simulink model "HVModAL_Fahrzeugmodell"  (R2015b)
settings: Solver=ode1  StartTime=0  StopTime=drp.driving_cycle.tstop  FixedStep=sim_params.Ts  RelTol=1e-5
PreLoadFcn:
  | % Add paths
  | addpath data
  | addpath(genpath('library'))
StartFcn:
  | Simulation.StartTime = tic;
StopFcn:
  | Simulation.DurationTime = toc(Simulation.StartTime);
undefined symbols (not defined in the file or in its folder): Batteries, BMS, BMS_Bat_, C_Nenn_DCDC1, C_Nenn_DCDC2, d2d, DC, DCDC_Converter_efficiency, DcDc_Converters, Dcl, drp, drv, elm, gen, gin, Hdc, hdc, HV, hvb, Hvb, ice, ldc, lib_dcl, lib_hdc, lib_hvb, lib_veh, Link, lossestable, mask_LUT_OCV, mask_LUT_OCV_SOC, mask_LUT_OCV_Temperature, mask_LUT_R, mask_LUT_Rs, mask_LUT_Rs_SOC, mask_LUT_Rs_Temperature, sim_params, speedvec, torquevec, tri, veh, Veh, Vehicle_Chassis
libraries: simulink x29, lib_tri_modules x7, lib_hdc_module x5, lib_gearbox x4, lib_hvb_battery_pack x3, cstblocks x3, PowerLimitBlock x2, MultiCellLibrary x2, lib_aux x1, lib_drv x1, lib_gen x1, lib_elm x1
(part 6 of 7)

== system HVModAL_Fahrzeugmodell/Energy Manager (Emg)/Battery Control/Driving_Mode/Strategy_Maximiziation_Available_Batterypower/Choice_Algorithm ==
  b_Bat_available_b_Bat1 : Inport
  b_Bat_available_b_Bat2 : Inport  Port=2
  b_Bat_available_b_Bat3 : Inport  Port=3
  n_Bat_type_ID_Bat1 : Inport  Port=4
  n_Bat_type_ID_Bat2 : Inport  Port=5
  n_Bat_type_ID_Bat3 : Inport  Port=6
  1_eq_2 : RelationalOperator  Operator===  OutDataTypeStr=boolean
  1_eq_3 : RelationalOperator  Operator===  OutDataTypeStr=boolean
  1av_AND_2av_AND_3av_AND_1_eq_2_eq3 : Logic  Inputs=6  AllPortsSameDT=off  OutDataTypeStr=boolean
  1av_AND_2av_AND_3not_av_AND_1_eq_2 : Logic  Inputs=4  AllPortsSameDT=off  OutDataTypeStr=boolean
  1av_AND_2not_av_AND_3av_AND_1_eq_3 : Logic  Inputs=4  AllPortsSameDT=off  OutDataTypeStr=boolean
  1not_av_AND_2av_AND_3av_AND_2_eq_3 : Logic  Inputs=4  AllPortsSameDT=off  OutDataTypeStr=boolean
  2_eq_3 : RelationalOperator  Operator===  OutDataTypeStr=boolean
  Logical Operator : Logic  Operator=NOT  AllPortsSameDT=off  OutDataTypeStr=boolean
  Logical Operator1 : Logic  Operator=NOT  AllPortsSameDT=off  OutDataTypeStr=boolean
  Logical Operator2 : Logic  Operator=NOT  AllPortsSameDT=off  OutDataTypeStr=boolean
  Logical Operator3 : Logic  Operator=OR  Inputs=4  AllPortsSameDT=off  OutDataTypeStr=boolean
  b_Strategy_SOC_Equalization : Outport
  wires:
  Logical Operator3/1 -> b_Strategy_SOC_Equalization/1
  1av_AND_2not_av_AND_3av_AND_1_eq_3/1 -> Logical Operator3/3
  1av_AND_2av_AND_3not_av_AND_1_eq_2/1 -> Logical Operator3/2
  1not_av_AND_2av_AND_3av_AND_2_eq_3/1 -> Logical Operator3/4
  1av_AND_2av_AND_3av_AND_1_eq_2_eq3/1 -> Logical Operator3/1
  Logical Operator2/1 -> 1not_av_AND_2av_AND_3av_AND_2_eq_3/1
  Logical Operator1/1 -> 1av_AND_2not_av_AND_3av_AND_1_eq_3/2
  Logical Operator/1 -> 1av_AND_2av_AND_3not_av_AND_1_eq_2/3
  1_eq_3/1 -> 1av_AND_2not_av_AND_3av_AND_1_eq_3/4, 1av_AND_2av_AND_3av_AND_1_eq_2_eq3/6
  2_eq_3/1 -> 1av_AND_2av_AND_3av_AND_1_eq_2_eq3/5, 1not_av_AND_2av_AND_3av_AND_2_eq_3/4
  1_eq_2/1 -> 1av_AND_2av_AND_3not_av_AND_1_eq_2/4, 1av_AND_2av_AND_3av_AND_1_eq_2_eq3/4
  n_Bat_type_ID_Bat3/1 -> 2_eq_3/2, 1_eq_3/2
  n_Bat_type_ID_Bat2/1 -> 1_eq_2/2, 2_eq_3/1
  n_Bat_type_ID_Bat1/1 -> 1_eq_2/1, 1_eq_3/1
  b_Bat_available_b_Bat3/1 -> Logical Operator/1, 1av_AND_2av_AND_3av_AND_1_eq_2_eq3/3, 1av_AND_2not_av_AND_3av_AND_1_eq_3/3, 1not_av_AND_2av_AND_3av_AND_2_eq_3/3
  b_Bat_available_b_Bat2/1 -> 1av_AND_2av_AND_3not_av_AND_1_eq_2/2, 1av_AND_2av_AND_3av_AND_1_eq_2_eq3/2, Logical Operator1/1, 1not_av_AND_2av_AND_3av_AND_2_eq_3/2
  b_Bat_available_b_Bat1/1 -> Logical Operator2/1, 1av_AND_2not_av_AND_3av_AND_1_eq_3/1, 1av_AND_2av_AND_3not_av_AND_1_eq_2/1, 1av_AND_2av_AND_3av_AND_1_eq_2_eq3/1

== system HVModAL_Fahrzeugmodell/Energy Manager (Emg)/Battery Control/Driving_Mode/Strategy_Maximiziation_Available_Batterypower/multiple_packs ==
  b_Bat_available_b_Bat1 : Inport
  b_Bat_available_b_Bat2 : Inport  Port=2
  b_Bat_available_b_Bat3 : Inport  Port=3
  Add : Sum  Inputs=+++
  Constant : Constant
  Display : Display
  Relational Operator : RelationalOperator  Operator=>  OutDataTypeStr=boolean
  b_MultiplePacks : Outport
  wires:
  b_Bat_available_b_Bat1/1 -> Add/1
  b_Bat_available_b_Bat2/1 -> Add/2
  b_Bat_available_b_Bat3/1 -> Add/3
  Add/1 -> Display/1, Relational Operator/1
  Constant/1 -> Relational Operator/2
  Relational Operator/1 -> b_MultiplePacks/1

== system HVModAL_Fahrzeugmodell/Energy Manager (Emg)/Battery Control/Driving_Mode/Strategy_Maximiziation_Available_Batterypower/only_one_Pack ==
  note: full power to available pack
  b_Bat_available_b_Bat1 : Inport
  b_Bat_available_b_Bat2 : Inport  Port=2
  b_Bat_available_b_Bat3 : Inport  Port=3
  Enable : EnablePort
  Gain : Gain  Gain=100
  Gain1 : Gain  Gain=100
  Gain2 : Gain  Gain=100
  Mux : Mux  Inputs=3
  vector_PowerDistribution : Outport
  wires:
  b_Bat_available_b_Bat1/1 -> Gain/1
  b_Bat_available_b_Bat2/1 -> Gain1/1
  b_Bat_available_b_Bat3/1 -> Gain2/1
  Mux/1 -> vector_PowerDistribution/1
  Gain/1 -> Mux/1
  Gain1/1 -> Mux/2
  Gain2/1 -> Mux/3

== system HVModAL_Fahrzeugmodell/Energy Manager (Emg)/Battery Control/Driving_Mode/Strategy_Maximiziation_Driving_Range1/Minloss Strategy ==
  SB_BMS_1 : Inport
  SB_BMS_2 : Inport  Port=2
  SB_BMS_3 : Inport  Port=3
  Pload : Inport  Port=4
  Bus Selector : BusSelector  OutputSignals=SOC_perc
  Compare To Constant : simulink/Logic and Bit Operations/Compare To Constant  relop=>=  const=20  OutDataTypeStr=boolean
  Insufficient Energy : Subsystem
  Logical Operator : Logic  Operator=NOT  AllPortsSameDT=off  OutDataTypeStr=boolean
  Merge : Merge
  Merge1 : Merge
  Sufficient Energy left : Subsystem
  vector_PowerDistribution : Outport
  P_exchange_Master_Slave : Outport  Port=2
  wires:
  Insufficient Energy/2(P_exchange_Master_Slave) -> Merge1/2
  Sufficient Energy left/2(P_exchange_Master_Slave) -> Merge1/1
  Merge1/1 -> P_exchange_Master_Slave/1
  Logical Operator/1 -> Insufficient Energy/Enable
  Merge/1 -> vector_PowerDistribution/1
  Insufficient Energy/1(vector_PowerDistribution) -> Merge/2
  Sufficient Energy left/1(vector_PowerDistribution) -> Merge/1
  Compare To Constant/1 -> Logical Operator/1, Sufficient Energy left/Enable
  Bus Selector/1 -> Compare To Constant/1  "<SOC_perc>"
  Pload/1 -> Sufficient Energy left/4(Pload), Insufficient Energy/4("Pload ")
  SB_BMS_3/1 -> Insufficient Energy/3("SB_BMS_3 "), Sufficient Energy left/3("SB_BMS_3 ")
  SB_BMS_2/1 -> Insufficient Energy/2(SB_BMS_2), Sufficient Energy left/2(SB_BMS_2)
  SB_BMS_1/1 -> Bus Selector/1, Insufficient Energy/1(SB_BMS_1), Sufficient Energy left/1(SB_BMS_1)

== system HVModAL_Fahrzeugmodell/Traction Inverters (Tri)/Tri1/Thermal Model/Conventional thermal model/Conventional thermal model ==
  P losses : Inport
  T_amb : Inport  Port=2
  Demux1 : Demux
  Mux3 : Mux
  Subsystem : Subsystem
  Temperature : Outport
  wires:
  Demux1/3 -> Subsystem/3(Ploss Ml)
  Demux1/2 -> Subsystem/2(Ploss Dh)
  Demux1/1 -> Subsystem/1(Ploss Mh)
  P losses/1 -> Demux1/1
  Demux1/4 -> Subsystem/4(Ploss Dl)
  T_amb/1 -> Subsystem/5(Water Temperature)
  Mux3/1 -> Temperature/1
  Subsystem/4(T Dl) -> Mux3/4
  Subsystem/3(T Ml) -> Mux3/3
  Subsystem/1(T Mh) -> Mux3/1
  Subsystem/2(T Dh) -> Mux3/2

== system HVModAL_Fahrzeugmodell/Traction Inverters (Tri)/Tri1/Thermal Model/Foster Model/Leg1 ==
  In1 : Inport
  Constant : Constant  Value=TRIname.ThermalModel.FosterModel.FosterModel.IGBT.firstValue
  Constant1 : Constant  Value=[TRIname.ThermalModel.FosterModel.FosterModel.Diode.firstValue]
  Constant2 : Constant  Value=[TRIname.ThermalModel.FosterModel.FosterModel.IGBT.firstValue]
  Constant3 : Constant  Value=[TRIname.ThermalModel.FosterModel.FosterModel.Diode.firstValue]
  Demux : Demux
  Mux : Mux
  Product{,1..3} (4 alike) : Product
  Sum{1..6,16,18} (8 alike) : Sum  Inputs=|++
  Transfer Fcn1 : TransferFcn  Numerator=[TRIname.ThermalModel.FosterModel.FosterModel.IGBT.secondValue]  Denominator=[TRIname.ThermalModel.FosterModel.FosterModel.IGBT.secondTau 1]
  Transfer Fcn2 : TransferFcn  Numerator=[TRIname.ThermalModel.FosterModel.FosterModel.IGBT.transientValue]  Denominator=[TRIname.ThermalModel.FosterModel.FosterModel.IGBT.transientTau 1]
  Transfer Fcn3 : TransferFcn  Numerator=[TRIname.ThermalModel.FosterModel.FosterModel.Diode.secondValue]  Denominator=[TRIname.ThermalModel.FosterModel.FosterModel.Diode.secondTau 1]
  Transfer Fcn4 : TransferFcn  Numerator=[TRIname.ThermalModel.FosterModel.FosterModel.Diode.transientValue]  Denominator=[TRIname.ThermalModel.FosterModel.FosterModel.Diode.transientTau 1]
  Transfer Fcn5 : TransferFcn  Numerator=[TRIname.ThermalModel.FosterModel.FosterModel.IGBT.secondValue]  Denominator=[TRIname.ThermalModel.FosterModel.FosterModel.IGBT.secondTau 1]
  Transfer Fcn6 : TransferFcn  Numerator=[TRIname.ThermalModel.FosterModel.FosterModel.IGBT.transientValue]  Denominator=[TRIname.ThermalModel.FosterModel.FosterModel.IGBT.transientTau 1]
  Transfer Fcn7 : TransferFcn  Numerator=[TRIname.ThermalModel.FosterModel.FosterModel.Diode.secondValue]  Denominator=[TRIname.ThermalModel.FosterModel.FosterModel.Diode.secondTau 1]
  Transfer Fcn8 : TransferFcn  Numerator=[TRIname.ThermalModel.FosterModel.FosterModel.Diode.transientValue]  Denominator=[TRIname.ThermalModel.FosterModel.FosterModel.Diode.transientTau 1]
  Leg1TempVec : Outport
  wires:
  Sum6/1 -> Mux/4
  Product2/1 -> Sum4/1
  Transfer Fcn5/1 -> Sum4/2
  Constant2/1 -> Product2/1
  Transfer Fcn8/1 -> Sum6/2
  Transfer Fcn7/1 -> Sum3/2
  Product3/1 -> Sum3/1
  Transfer Fcn6/1 -> Sum5/2
  Sum3/1 -> Sum6/1
  Sum4/1 -> Sum5/1
  Constant3/1 -> Product3/1
  Sum5/1 -> Mux/3
  Demux/3 -> Product2/2, Transfer Fcn5/1, Transfer Fcn6/1
  Demux/4 -> Transfer Fcn8/1, Transfer Fcn7/1, Product3/2
  Mux/1 -> Leg1TempVec/1
  In1/1 -> Demux/1
  Sum1/1 -> Sum2/1
  Demux/2 -> Product1/2, Transfer Fcn3/1, Transfer Fcn4/1
  Constant1/1 -> Product1/1
  Sum2/1 -> Mux/2
  Transfer Fcn4/1 -> Sum2/2
  Product1/1 -> Sum1/1
  Transfer Fcn3/1 -> Sum1/2
  Constant/1 -> Product/1
  Sum18/1 -> Mux/1
  Sum16/1 -> Sum18/1
  Demux/1 -> Transfer Fcn2/1, Transfer Fcn1/1, Product/2
  Transfer Fcn2/1 -> Sum18/2
  Product/1 -> Sum16/1
  Transfer Fcn1/1 -> Sum16/2

== system HVModAL_Fahrzeugmodell/Traction Inverters (Tri)/Tri1/Thermal Model old/Thermal Junction Model/Leg 1 ==
  In1 : Inport
  Leg 1_sfcn : S-Function  FunctionName=Leg_sf  SFunctionModules=""  SFunctionDeploymentMode=off  EnableBusSupport=off  mask{rtw_sf_name=Leg_sf, showVar=off}
      mask prompts: rtw_sf_name "Simulink:masks:GenSFuncName_MP"; showVar "Simulink:masks:GenSFuncShowModuleList_MP"
      mask help: Simulink:masks:GenSFuncDesc_MD
      mask init: same as HVModAL_Fahrzeugmodell/Energy Manager (Emg)/Battery Control1/Battery Control_sfcn
      settings: CopyFcn=|
      | if ~strcmp(get_param(gcb,'Linkstatus'),'none') && ...
      | ~strcmp(get_param(gcb,'Linkstatus'),'implicit')
      |   set_param(gcb,'LinkStatus','none');
      | end
      mask Help: eval('feval(''rtwprivate'',''rtwhelpview'',''rtw_sfcn_block'')');
      mask Display:
      | port_label('input',1,'In1');
      | port_label('output',1,'Out1');
  __InputSSForSFun__ : Subsystem
      settings: PermitHierarchicalResolution=ParametersOnly
  __OutputSSForSFun__ : Subsystem
      settings: PermitHierarchicalResolution=ParametersOnly
  Out1 : Outport  InitialOutput=0
  wires:
  __OutputSSForSFun__/1(Out1) -> Out1/1
  Leg 1_sfcn/1 -> __OutputSSForSFun__/1(__UniqueInportName__1__)
  __InputSSForSFun__/1(__UniqueOutportName__1__) -> Leg 1_sfcn/1
  In1/1 -> __InputSSForSFun__/1(In1)

== system HVModAL_Fahrzeugmodell/Traction Inverters (Tri)/Tri1/Thermal Model old/Thermal Junction Model/Leg 2 ==
  In1 : Inport
  Leg 1_sfcn : S-Function  FunctionName=Leg_sf  SFunctionModules=""  SFunctionDeploymentMode=off  EnableBusSupport=off  mask{rtw_sf_name=Leg_sf, showVar=off}
      mask prompts: rtw_sf_name "Simulink:masks:GenSFuncName_MP"; showVar "Simulink:masks:GenSFuncShowModuleList_MP"
      mask help: Simulink:masks:GenSFuncDesc_MD
      mask init: same as HVModAL_Fahrzeugmodell/Energy Manager (Emg)/Battery Control1/Battery Control_sfcn
      settings: CopyFcn=|
      | if ~strcmp(get_param(gcb,'Linkstatus'),'none') && ...
      | ~strcmp(get_param(gcb,'Linkstatus'),'implicit')
      |   set_param(gcb,'LinkStatus','none');
      | end
      mask Help: eval('feval(''rtwprivate'',''rtwhelpview'',''rtw_sfcn_block'')');
      mask Display:
      | port_label('input',1,'In1');
      | port_label('output',1,'Out1');
  __InputSSForSFun__ : Subsystem
      settings: PermitHierarchicalResolution=ParametersOnly
  __OutputSSForSFun__ : Subsystem
      settings: PermitHierarchicalResolution=ParametersOnly
  Out1 : Outport  InitialOutput=0
  wires:
  __OutputSSForSFun__/1(Out1) -> Out1/1
  Leg 1_sfcn/1 -> __OutputSSForSFun__/1(__UniqueInportName__1__)
  __InputSSForSFun__/1(__UniqueOutportName__1__) -> Leg 1_sfcn/1
  In1/1 -> __InputSSForSFun__/1(In1)

== system HVModAL_Fahrzeugmodell/Traction Inverters (Tri)/Tri1/Thermal Model old/Thermal Junction Model/Leg 3 ==
  In1 : Inport
  Leg 1_sfcn : S-Function  FunctionName=Leg_sf  SFunctionModules=""  SFunctionDeploymentMode=off  EnableBusSupport=off  mask{rtw_sf_name=Leg_sf, showVar=off}
      mask prompts: rtw_sf_name "Simulink:masks:GenSFuncName_MP"; showVar "Simulink:masks:GenSFuncShowModuleList_MP"
      mask help: Simulink:masks:GenSFuncDesc_MD
      mask init: same as HVModAL_Fahrzeugmodell/Energy Manager (Emg)/Battery Control1/Battery Control_sfcn
      settings: CopyFcn=|
      | if ~strcmp(get_param(gcb,'Linkstatus'),'none') && ...
      | ~strcmp(get_param(gcb,'Linkstatus'),'implicit')
      |   set_param(gcb,'LinkStatus','none');
      | end
      mask Help: eval('feval(''rtwprivate'',''rtwhelpview'',''rtw_sfcn_block'')');
      mask Display:
      | port_label('input',1,'In1');
      | port_label('output',1,'Out1');
  __InputSSForSFun__ : Subsystem
      settings: PermitHierarchicalResolution=ParametersOnly
  __OutputSSForSFun__ : Subsystem
      settings: PermitHierarchicalResolution=ParametersOnly
  Out1 : Outport  InitialOutput=0
  wires:
  In1/1 -> __InputSSForSFun__/1(In1)
  __InputSSForSFun__/1(__UniqueOutportName__1__) -> Leg 1_sfcn/1
  Leg 1_sfcn/1 -> __OutputSSForSFun__/1(__UniqueInportName__1__)
  __OutputSSForSFun__/1(Out1) -> Out1/1

== system HVModAL_Fahrzeugmodell/Energy Manager (Emg)/Battery Control/Driving_Mode/Range_extender 1/power_distribution_new/Subsystem ==
  note: #new#:
      | P_load-P_Bat2_max>0: --> P_load>P_Bat2_max --> P2=P_Bat2_max; P1=P_load-P2; discharge
      |
      | P_load-P_Bat2_max<0: --> 1): 0<P_load<P_Bat2_max -->P2=P_load*3; P1=P_load-P2; charged or (0<P_load<P_Bat2_max -->P2=P_load; P1=0;)
      |
      | 2): P_load<0 --> P2=|P_load|&P2<=P_Bat2_max; P1=P_load+P2; charged
  note: #previous#:
      | P_load-P_Bat2_max>0: --> P_load>P_Bat2_max --> P2=P_Bat2_max; P1=P_load-P2; discharge
      |
      | P_load-P_Bat2_max<0: --> 1): 0<P_load<P_Bat2_max -->P2=P_Bat2_max; P1=P_load-P2; charged
      |
      | 2): P_load<0 --> P2=P_Bat2_max; P1=P_load+P2; charged
  P_load : Inport
  P_Bat2_discharge_max : Inport  Port=2
  Constant1 : Constant  Value=0
  Gain : Gain  Gain=-1
  Gain1 : Gain  Gain=3
  P_Bat2_new : Scope  NumInputPorts=2
  P_Bat2_old : Scope  NumInputPorts=2
  P_UB_Bat1#2 : Scope
  Saturation1 : Saturate  UpperLimit=0  LowerLimit=-inf
  Subtract1 : Sum  Inputs=+-
  Subtract2 : Sum  Inputs=+-
  Subtract3 : Sum  Inputs=+-
  Switch{1,3..5} (4 alike) : Switch
  Switch2 : Switch  Threshold=5
  P_Bat2 : Outport
  wires:
  Switch1/1 -> P_Bat2/1, P_Bat2_new/2
  P_Bat2_discharge_max/1 -> Subtract2/2, Switch5/1, P_UB_Bat1#2/1, Switch1/1, Subtract3/2, Switch2/1
  Constant1/1 -> Switch2/3
  Switch2/1 -> Subtract1/2, Switch3/1
  Subtract1/1 -> Switch3/2
  Switch3/1 -> Switch4/1, Switch4/2
  Saturation1/1 -> Gain/1
  Gain/1 -> Switch5/3, Subtract2/1
  Subtract2/1 -> Switch5/2
  Switch5/1 -> Switch4/3
  Subtract3/1 -> Switch1/2
  Gain1/1 -> Switch1/3, Subtract3/1
  Switch4/1 -> P_Bat2_old/2, Gain1/1
  P_load/1 -> Switch2/2, Saturation1/1, Switch3/3, Subtract1/1, P_Bat2_new/1, P_Bat2_old/1

== system HVModAL_Fahrzeugmodell/Energy Manager (Emg)/Battery Control/Driving_Mode/Range_extender 2/dynamic/power estimination  ==
  note: pos. and negative
      | but != 0
  note: >0 --> Inverter take energy out of DC link (Acceleration)
      | <0 --> Inverter feed energy into DC link (Recuperation)
  note: calculate the voltage
  note: calculate the power
  P_max_Disch_W_Bat2 : Inport
  P_currentPower_W_Bat1 : Inport  Port=2
  P_currentPower_W_Bat2 : Inport  Port=3
  P_currentPower_W_Bat3 : Inport  Port=4
  P_max_ch_W_Bat1 : Inport  Port=5
  P_max_Disch_W_Bat1 : Inport  Port=6
  "I_rex " : Inport  Port=7
  P_currentPower_Inv_W : Inport  Port=8
  P_currentPower_Aux_W : Inport  Port=9
  Add1 : Sum
  Add2 : Sum  Inputs=+++
  Add3 : Sum
  Constant2 : Constant  Value=hvb.Bat2.cell.I_max_disch
  Constant3 : Constant  Value=0.1
  Divide1 : Product  Inputs=*/
  Gain : Gain  Gain=-1
  Gain1 : Gain
  Product1 : Product
  Scope1 : Scope  NumInputPorts=2
  Scope12 : Scope  NumInputPorts=2
  Switch : Switch  Criteria=u2 ~= 0  Threshold=0.5
  mapping1 : Subsystem  AncestorBlock=PowerDistribution_Dynamic_algo/Dynamic_power_distribution_1av_HE_AND_2av_HP/mapping1  TreatAsAtomicUnit=on
  p_bat2 : Outport
  P_Load_W : Outport  Port=2
  P_LB_Bat1 : Outport  Port=3
  P_UB_Bat1 : Outport  Port=4
  wires:
  Gain1/1 -> Add1/1, Switch/2, Switch/1
  Add1/1 -> Switch/3
  Constant3/1 -> Add1/2
  P_currentPower_W_Bat2/1 -> Add2/2
  Add2/1 -> Gain/1
  P_currentPower_W_Bat1/1 -> Add2/1
  P_currentPower_W_Bat3/1 -> Add2/3
  P_max_ch_W_Bat1/1 -> mapping1/1(P_max_ch_W_Bat1)
  P_max_Disch_W_Bat1/1 -> mapping1/2(P_max_Disch_W_Bat1)
  mapping1/1(P_LB_Bat1) -> P_LB_Bat1/1
  mapping1/2(P_UB_Bat1) -> P_UB_Bat1/1
  Switch/1 -> P_Load_W/1
  Constant2/1 -> Scope1/1, Divide1/2
  P_max_Disch_W_Bat2/1 -> Scope12/1, Divide1/1
  Divide1/1 -> Product1/1
  "I_rex "/1 -> Product1/2, Scope1/2
  Product1/1 -> Scope12/2, p_bat2/1
  P_currentPower_Inv_W/1 -> Add3/1
  P_currentPower_Aux_W/1 -> Add3/2
  Add3/1 -> Gain1/1

== system HVModAL_Fahrzeugmodell/Energy Manager (Emg)/Battery Control/Driving_Mode/Range_extender 2/dynamic/power_distribution_new ==
  note: entladen 3000
  note: rekuperieren: -10000
  note: entladen: 10000
  note: 0: highway mode (constant power strategy)
      | 1: city mode (power follow control strategy )
  P_Load_W : Inport
  P_UB_Bat1 : Inport  Port=2
  P_LB_Bat1 : Inport  Port=3
  Turn_on_range_extender : Inport  Port=4
  P_bat2_W : Inport  Port=5
  city_1_or_highway_0 : Inport  Port=6
  T_Cell_avg : Inport  Port=7
  Chart : Stateflow chart  TreatAsAtomicUnit=on
      settings: PermitHierarchicalResolution=ParametersOnly
  Constant2 : Constant  Value=0
  Mux : Mux  Inputs=3
  Product : Product
  Scope : Scope  NumInputPorts=2
  Subtract : Sum  Inputs=+-
  Switch2 : Switch  Criteria=u2 > Threshold
  abs2perc2 : Gain
  abs2perc3 : Gain
  abs2perc4 : Gain
  power_follow_control : Subsystem
  prevent_bat1_overcharge&& temperature control : Subsystem
  vector_PowerDistribution : Outport
  wires:
  Mux/1 -> vector_PowerDistribution/1
  abs2perc2/1 -> Mux/3  "PowerShare_Bat3"
  Constant2/1 -> abs2perc2/1
  P_LB_Bat1/1 -> Chart/3(P_LB_Bat1)
  P_UB_Bat1/1 -> Chart/2(P_UB_Bat1)
  Subtract/1 -> Chart/1(p_Bat1_o)
  Chart/1(P_Bat1) -> abs2perc3/1
  P_bat2_W/1 -> Product/1
  P_Load_W/1 -> prevent_bat1_overcharge&& temperature control/1("P_load "), Scope/1, Subtract/1, power_follow_control/1(P_load)
  Turn_on_range_extender/1 -> Product/2
  Product/1 -> Switch2/3, power_follow_control/2(P_Bat2_discharge_max)
  power_follow_control/1(P_Bat2) -> Switch2/1
  city_1_or_highway_0/1 -> Switch2/2
  abs2perc4/1 -> Mux/2
  abs2perc3/1 -> Mux/1
  Switch2/1 -> prevent_bat1_overcharge&& temperature control/2(P_bat2)
  prevent_bat1_overcharge&& temperature control/1("p_pat2_new ") -> Scope/2, abs2perc4/1, Subtract/2
  T_Cell_avg/1 -> prevent_bat1_overcharge&& temperature control/3(T_Cell_avg)

== system HVModAL_Fahrzeugmodell/Energy Manager (Emg)/Battery Control/Driving_Mode/Range_extender 2/dynamic/soc estimination  ==
  note: estimate whether driving range within the capability of the main battery(secondary battery
  note: soc<30 => soc=30
  note: soc>79 => soc=100
  note: soc > 79%             convert to 100% (small difference between the effects of step-in soc 100% and 80% )
      | 79% > soc > 30%  stay
      | 30% > soc              convert to 30% (step-in soc lower than 30%, I_rex will be too high, Bat2 will be consumed too fast )
  note: To determine the current in each cell (I_rex) and the step-in soc
      | by different bat1 capacity and driving range
  driving range : Inport
  soc_perc_01 : Inport  Port=2
  soc_perc_02 : Inport  Port=3
  bat1 : Inport  Port=4
  cell number : Inport  Port=5
  city or highway : Inport  Port=6
  Chart : Stateflow chart  TreatAsAtomicUnit=on
      settings: PermitHierarchicalResolution=ParametersOnly
  Chart3 : Stateflow chart  TreatAsAtomicUnit=on
      settings: PermitHierarchicalResolution=ParametersOnly
  Constant5 : Constant  Value=100
  Constant8 : Constant  Value=30
  Display : Display
  Display1 : Display
  Energy consumption pro km : Constant  Value=160
  Energy consumption pro km1 : Constant  Value=200
  Logical Operator3 : Logic  AllPortsSameDT=off  OutDataTypeStr=boolean
  Product2 : Product
  Relational Operator4 : RelationalOperator  Operator=<  OutDataTypeStr=boolean
  "SOC & I_rex " : Subsystem
  Saturation : Saturate  UpperLimit=hvb.Bat2.cell.I_max_disch  LowerLimit=0
  Scope{1..9,13} (10 alike) : Scope
  Scope14 : Scope  NumInputPorts=2
  Subtract : Sum  Inputs=+-
  Switch1 : Switch  Criteria=u2 > Threshold
  Switch2 : Switch  Criteria=u2 > Threshold
  Switch3 : Switch  Criteria=u2 > Threshold  Threshold=79
  Switch4 : Switch  Criteria=u2 > Threshold  Threshold=30
  constant : Constant
  everage speed : Constant  Value=50
  everage speed1 : Constant  Value=100
  specific energy consumption 160Wh/Km : Constant  Value=160
  "Turn_on_rex " : Outport
  I_rex 1 : Outport  Port=2
  wires:
  Chart/1(Use_Range_extender) -> [Use_range_extender], Scope3/1
  soc_perc_02/1 -> Chart/2(SOC_perc_02), Scope14/2
  soc_perc_01/1 -> Chart/1(SOC_perc_01), Scope14/1
  Relational Operator4/1 -> Scope1/1, [Enter_range_extender_mode]
  [Enter_range_extender_mode] -> Logical Operator3/1
  [Use_range_extender] -> Logical Operator3/2
  Logical Operator3/1 -> "Turn_on_rex "/1
  specific energy consumption 160Wh/Km/1 -> Product2/2
  Product2/1 -> Relational Operator4/2
  Energy consumption pro km/1 -> Switch2/1
  Switch4/1 -> [SOC], Scope4/1
  Saturation/1 -> Scope13/1, I_rex 1/1
  bat1/1 -> [bat1]
  [bat1] -> Relational Operator4/1
  driving range/1 -> [driving_range]
  [driving_range] -> Product2/1
  [SOC] -> Subtract/1
  constant/1 -> Subtract/2
  Subtract/1 -> Scope2/1, Chart/3(SOC_limit)
  city or highway/1 -> Switch2/2
  Energy consumption pro km1/1 -> Switch2/3
  everage speed/1 -> Switch1/1
  everage speed1/1 -> Switch1/3
  Constant5/1 -> Switch3/1
  Switch3/1 -> Switch4/1, Switch4/2
  Constant8/1 -> Switch4/3
  Switch1/1 -> Chart3/2(speed)
  Switch2/1 -> Chart3/3(E)
  Chart3/2(I_rex) -> Saturation/1
  Chart3/1(soc) -> Scope6/1, Switch3/3, Switch3/2
  Chart3/3(range) -> Scope7/1
  Chart3/4(range_2) -> Scope8/1
  Chart3/5(range_1) -> Scope9/1
  cell number/1 -> Display1/1, Chart3/4(cell)
  [bat1] -> Chart3/1(E_bat1), Scope5/1
  [driving_range] -> Display/1, Chart3/5(driving_range)

== system HVModAL_Fahrzeugmodell/Energy Manager (Emg)/Battery Control/Driving_Mode/Range_extender 2/start_from_30% 1/power estimination  ==
  note: vcltage
  note: pos. and negative
      | but != 0
  note: >0 --> Inverter take energy out of DC link (Acceleration)
      | <0 --> Inverter feed energy into DC link (Recuperation)
  P_currentPower_W_Bat1 : Inport
  P_currentPower_W_Bat2 : Inport  Port=2
  P_currentPower_W_Bat3 : Inport  Port=3
  P_max_ch_W_Bat1 : Inport  Port=4
  P_max_Disch_W_Bat1 : Inport  Port=5
  P_max_Disch_W_Bat2 : Inport  Port=6
  "I_rex " : Inport  Port=7
  P_currentPower_Inv_W : Inport  Port=8
  P_currentPower_Aux_W : Inport  Port=9
  Add1 : Sum
  Add2 : Sum  Inputs=+++
  Add3 : Sum
  Constant2 : Constant  Value=hvb.Bat2.cell.I_max_disch
  Constant3 : Constant  Value=0.1
  Divide1 : Product  Inputs=*/
  Gain : Gain
  Product1 : Product
  Scope12 : Scope  NumInputPorts=2
  Switch : Switch  Criteria=u2 ~= 0  Threshold=0.5
  mapping1 : Subsystem  AncestorBlock=PowerDistribution_Dynamic_algo/Dynamic_power_distribution_1av_HE_AND_2av_HP/mapping1  TreatAsAtomicUnit=on
  P_Load_W : Outport
  P_LB_Bat1 : Outport  Port=2
  P_UB_Bat1 : Outport  Port=3
  p_bat2 : Outport  Port=4
  wires:
  Gain/1 -> Add1/1, Switch/2, Switch/1
  Add1/1 -> Switch/3
  Constant3/1 -> Add1/2
  P_currentPower_W_Bat2/1 -> Add2/2
  Add2/1 -> ?
  P_currentPower_W_Bat1/1 -> Add2/1
  P_currentPower_W_Bat3/1 -> Add2/3
  P_max_ch_W_Bat1/1 -> mapping1/1(P_max_ch_W_Bat1)
  P_max_Disch_W_Bat1/1 -> mapping1/2(P_max_Disch_W_Bat1)
  mapping1/1(P_LB_Bat1) -> P_LB_Bat1/1
  mapping1/2(P_UB_Bat1) -> P_UB_Bat1/1
  Switch/1 -> P_Load_W/1
  Constant2/1 -> Divide1/2
  P_max_Disch_W_Bat2/1 -> Scope12/1, p_bat2/1, Divide1/1
  Divide1/1 -> Product1/1
  "I_rex "/1 -> Product1/2
  Product1/1 -> Scope12/2
  P_currentPower_Inv_W/1 -> Add3/2
  P_currentPower_Aux_W/1 -> Add3/1
  Add3/1 -> Gain/1

== system HVModAL_Fahrzeugmodell/Energy Manager (Emg)/Battery Control/Driving_Mode/Range_extender 2/start_from_30% 1/power_distribution_new ==
  note: entladen 3000
  note: rekuperieren: -10000
  note: entladen: 10000
  P_Load_W : Inport
  P_UB_Bat1 : Inport  Port=2
  P_LB_Bat1 : Inport  Port=3
  Turn_on_range_extender : Inport  Port=4
  P_discharge_W : Inport  Port=5
  T_Cell_avg : Inport  Port=6
  Chart : Stateflow chart  TreatAsAtomicUnit=on
      settings: PermitHierarchicalResolution=ParametersOnly
  Constant2 : Constant  Value=0
  Mux : Mux  Inputs=3
  Product : Product
  Subtract : Sum  Inputs=+-
  abs2perc2 : Gain
  abs2perc3 : Gain
  abs2perc4 : Gain
  prevent_bat1_overcharge&& temperature control : Subsystem
  vector_PowerDistribution : Outport
  wires:
  Mux/1 -> vector_PowerDistribution/1
  abs2perc2/1 -> Mux/3  "PowerShare_Bat3"
  Constant2/1 -> abs2perc2/1
  P_LB_Bat1/1 -> Chart/3(P_LB_Bat1)
  P_UB_Bat1/1 -> Chart/2(P_UB_Bat1)
  Subtract/1 -> Chart/1(p_Bat1_o)
  Chart/1(P_Bat1) -> abs2perc3/1
  P_discharge_W/1 -> Product/1
  P_Load_W/1 -> prevent_bat1_overcharge&& temperature control/1("p_load "), Subtract/1
  Turn_on_range_extender/1 -> Product/2
  abs2perc4/1 -> Mux/2
  abs2perc3/1 -> Mux/1
  Product/1 -> prevent_bat1_overcharge&& temperature control/2(p_bat2_previous)
  prevent_bat1_overcharge&& temperature control/1("p_pat2_now ") -> Subtract/2, abs2perc4/1
  T_Cell_avg/1 -> prevent_bat1_overcharge&& temperature control/3(T_Cell_avg)

== system HVModAL_Fahrzeugmodell/Energy Manager (Emg)/Battery Control/Driving_Mode/Range_extender 2/start_from_30% 1/soc estimination  ==
  note: estimate whether driving range within the capability of the main battery(secondary battery
  note: rest=soc*E_bat1/100;...
      |  range_1=rest/E;....
      |  t=range_1/speed;...
      |  I_rex=3.1/t;...
  soc_perc_01 : Inport
  soc_perc_02 : Inport  Port=2
  bat1 : Inport  Port=3
  driving range : Inport  Port=4
  Veh_v_actual : Inport  Port=5
  city_1_or_highway_0 : Inport  Port=6
  Chart : Stateflow chart  TreatAsAtomicUnit=on
      settings: PermitHierarchicalResolution=ParametersOnly
  Constant1 : Constant  Value=30
  Constant10 : Constant  Value=3.1
  Constant2 : Constant  Value=30
  Constant9 : Constant  Value=100
  Divide2 : Product  Inputs=**///
  Divide3 : Product  Inputs=*/
  Energy consumption pro km : Constant  Value=160
  Energy consumption pro km1 : Constant  Value=200
  Logical Operator3 : Logic  AllPortsSameDT=off  OutDataTypeStr=boolean
  Product2 : Product
  Relational Operator4 : RelationalOperator  Operator=<  OutDataTypeStr=boolean
  Saturation : Saturate  UpperLimit=3  LowerLimit=0
  Scope{1,3..4,13} (4 alike) : Scope
  Scope14 : Scope  NumInputPorts=2
  Subsystem : Subsystem
  Switch1 : Switch  Criteria=u2 > Threshold
  Switch2 : Switch  Criteria=u2 > Threshold
  everage speed : Constant  Value=50
  everage speed1 : Constant  Value=100
  specific energy consumption 160Wh/Km : Constant  Value=160
  "Turn_on_rex " : Outport
  I_rex 1 : Outport  Port=2
  tag scope: Use_Range_extender=global
  wires:
  Chart/1(Use_Range_extender) -> Scope3/1, [Use_Range_extender]
  soc_perc_01/1 -> Chart/1(SOC_perc_01), Scope14/1, Subsystem/1(soc_perc_bat1)
  [Enter_range_extender_mode] -> Logical Operator3/1
  [Use_Range_extender] -> Logical Operator3/2
  Logical Operator3/1 -> Scope1/1, "Turn_on_rex "/1
  Constant1/1 -> Chart/3(SOC_limit)
  Relational Operator4/1 -> [Enter_range_extender_mode]
  specific energy consumption 160Wh/Km/1 -> Product2/2
  Product2/1 -> Relational Operator4/2
  bat1/1 -> [bat1]
  [bat1] -> Relational Operator4/1
  driving range/1 -> [driving_range]
  [driving_range] -> Product2/1
  soc_perc_02/1 -> Scope14/2, Chart/2(SOC_perc_02)
  [bat1] -> Subsystem/2(E_bat1)
  [driving_range] -> Subsystem/3(driving_range)
  Veh_v_actual/1 -> Subsystem/4(V)
  Subsystem/1(only_bat1_capability) -> Chart/4(only_bat1_capability)
  Divide2/1 -> Divide3/2
  Constant9/1 -> Divide2/3
  Divide3/1 -> Saturation/1
  Constant10/1 -> Divide3/1
  Switch1/1 -> Divide2/5
  Switch2/1 -> Divide2/4
  [bat1] -> Divide2/2
  Saturation/1 -> I_rex 1/1, Scope13/1
  Constant2/1 -> [SOC], Scope4/1, Divide2/1
  Energy consumption pro km/1 -> Switch2/1
  city_1_or_highway_0/1 -> Switch1/2, Switch2/2
  Energy consumption pro km1/1 -> Switch2/3
  everage speed/1 -> Switch1/1
  everage speed1/1 -> Switch1/3

== system HVModAL_Fahrzeugmodell/Energy Manager (Emg)/Battery Control/Driving_Mode/Range_extender 2/start_from_begining /power estimination  ==
  note: calculate the voltage
  note: calculate the power
  note: pos. and negative
      | but != 0
  note: >0 --> Inverter take energy out of DC link (Acceleration)
      | <0 --> Inverter feed energy into DC link (Recuperation)
  P_max_ch_W_Bat1 : Inport
  P_max_Disch_W_Bat1 : Inport  Port=2
  P_max_Disch_W_Bat2 : Inport  Port=3
  "I_rex " : Inport  Port=4
  P_currentPower_Inv_W : Inport  Port=5
  P_currentPower_Aux_W : Inport  Port=6
  Add1 : Sum
  Add3 : Sum
  Constant2 : Constant  Value=hvb.Bat2.cell.I_max_disch
  Constant3 : Constant  Value=0.1
  Divide1 : Product  Inputs=*/
  Gain : Gain
  Product1 : Product
  Scope12 : Scope  NumInputPorts=2
  Switch : Switch  Criteria=u2 ~= 0  Threshold=0.5
  mapping1 : Subsystem  AncestorBlock=PowerDistribution_Dynamic_algo/Dynamic_power_distribution_1av_HE_AND_2av_HP/mapping1  TreatAsAtomicUnit=on
  P_LB_Bat1 : Outport
  P_UB_Bat1 : Outport  Port=2
  p_bat2 : Outport  Port=3
  P_Load_W : Outport  Port=4
  wires:
  P_max_ch_W_Bat1/1 -> mapping1/1(P_max_ch_W_Bat1)
  P_max_Disch_W_Bat1/1 -> mapping1/2(P_max_Disch_W_Bat1)
  mapping1/1(P_LB_Bat1) -> P_LB_Bat1/1
  mapping1/2(P_UB_Bat1) -> P_UB_Bat1/1
  Constant2/1 -> Divide1/2
  P_max_Disch_W_Bat2/1 -> Scope12/1, Divide1/1
  Divide1/1 -> Product1/1
  "I_rex "/1 -> Product1/2
  Product1/1 -> p_bat2/1, Scope12/2
  Gain/1 -> Add1/1, Switch/2, Switch/1
  Add1/1 -> Switch/3
  Constant3/1 -> Add1/2
  Switch/1 -> P_Load_W/1
  P_currentPower_Inv_W/1 -> Add3/2
  P_currentPower_Aux_W/1 -> Add3/1
  Add3/1 -> Gain/1

== system HVModAL_Fahrzeugmodell/Energy Manager (Emg)/Battery Control/Driving_Mode/Range_extender 2/start_from_begining /power_distribution_new ==
  note: entladen 3000
  note: rekuperieren: -10000
  note: entladen: 10000
  note: 0: highway mode (constant power strategy)
      | 1: city mode (power follow control strategy )
  P_Load_W : Inport
  P_UB_Bat1 : Inport  Port=2
  P_LB_Bat1 : Inport  Port=3
  Turn_on_range_extender : Inport  Port=4
  P_discharge_W : Inport  Port=5
  city_1_or_highway_0 : Inport  Port=6
  T_Cell_avg : Inport  Port=7
  Chart : Stateflow chart  TreatAsAtomicUnit=on
      settings: PermitHierarchicalResolution=ParametersOnly
  Constant2 : Constant  Value=0
  Mux : Mux  Inputs=3
  Product : Product
  Subtract : Sum  Inputs=+-
  Switch2 : Switch  Criteria=u2 > Threshold
  abs2perc2 : Gain
  abs2perc3 : Gain
  abs2perc4 : Gain
  power_follow_control : Subsystem
  prevent_bat1_overcharge&& temperature control : Subsystem
  vector_PowerDistribution : Outport
  wires:
  Mux/1 -> vector_PowerDistribution/1
  abs2perc2/1 -> Mux/3  "PowerShare_Bat3"
  Constant2/1 -> abs2perc2/1
  P_LB_Bat1/1 -> Chart/3(P_LB_Bat1)
  P_UB_Bat1/1 -> Chart/2(P_UB_Bat1)
  Subtract/1 -> Chart/1(p_Bat1_o)
  Chart/1(P_Bat1) -> abs2perc3/1
  P_discharge_W/1 -> Product/1
  P_Load_W/1 -> prevent_bat1_overcharge&& temperature control/1("p_load "), Subtract/1, power_follow_control/1(P_load)
  Turn_on_range_extender/1 -> Product/2
  Product/1 -> Switch2/3, power_follow_control/2(P_Bat2_discharge_max)
  power_follow_control/1(P_Bat2) -> Switch2/1
  city_1_or_highway_0/1 -> Switch2/2
  abs2perc4/1 -> Mux/2
  abs2perc3/1 -> Mux/1
  Switch2/1 -> prevent_bat1_overcharge&& temperature control/2(p_bat2_old)
  prevent_bat1_overcharge&& temperature control/1("p_pat2_new ") -> Subtract/2, abs2perc4/1
  T_Cell_avg/1 -> prevent_bat1_overcharge&& temperature control/3(T_Cell_avg)

== system HVModAL_Fahrzeugmodell/Energy Manager (Emg)/Battery Control/Driving_Mode/Range_extender 2/start_from_begining /soc estimination  ==
  note: estimate whether driving range within the capability of the main battery(secondary battery
  note: rest=soc*E_bat1/100;...
      |  range_1=rest/E;....
      |  t=range_1/speed;...
      |  I_rex=3.1/t;...
  soc_perc_01 : Inport
  soc_perc_02 : Inport  Port=2
  bat1 : Inport  Port=3
  driving range : Inport  Port=4
  city_1_or_highway_0 : Inport  Port=5
  Chart : Stateflow chart  TreatAsAtomicUnit=on
      settings: PermitHierarchicalResolution=ParametersOnly
  Constant1 : Constant  Value=99
  Constant10 : Constant  Value=3.1
  Constant2 : Constant  Value=90
  Constant3 : Constant  Value=100
  Divide2 : Product  Inputs=**///
  Divide3 : Product  Inputs=*/
  Energy consumption pro km : Constant  Value=160
  Energy consumption pro km1 : Constant  Value=200
  Logical Operator3 : Logic  AllPortsSameDT=off  OutDataTypeStr=boolean
  Product1 : Product
  Relational Operator4 : RelationalOperator  Operator=<  OutDataTypeStr=boolean
  Saturation : Saturate  UpperLimit=hvb.Bat2.cell.I_max_disch  LowerLimit=0
  Scope{1..3,6,13} (5 alike) : Scope
  Scope14 : Scope  NumInputPorts=2
  Switch1 : Switch  Criteria=u2 > Threshold
  Switch2 : Switch  Criteria=u2 > Threshold
  everage speed : Constant  Value=50
  everage speed1 : Constant  Value=100
  specific energy consumption 160Wh/Km : Constant  Value=160
  "Turn_on_rex " : Outport
  I_rex 1 : Outport  Port=2
  wires:
  Chart/1(Use_Range_extender) -> [Use_Range_extender], Scope3/1
  soc_perc_02/1 -> Chart/2(SOC_perc_02), Scope14/2
  soc_perc_01/1 -> Chart/1(SOC_perc_01), Scope14/1
  [Enter_range_extender_mode] -> Logical Operator3/1
  [Use_Range_extender] -> Logical Operator3/2
  Logical Operator3/1 -> Scope1/1, "Turn_on_rex "/1
  Constant1/1 -> Scope2/1, Chart/3(SOC_limit)
  Relational Operator4/1 -> [Enter_range_extender_mode]
  driving range/1 -> Product1/1
  specific energy consumption 160Wh/Km/1 -> Product1/2
  Product1/1 -> Relational Operator4/2
  Energy consumption pro km/1 -> Switch2/1
  city_1_or_highway_0/1 -> Switch1/2, Switch2/2
  Energy consumption pro km1/1 -> Switch2/3
  Switch1/1 -> Divide2/5
  everage speed/1 -> Switch1/1
  everage speed1/1 -> Switch1/3
  Divide2/1 -> Divide3/2
  Switch2/1 -> Divide2/4
  Divide3/1 -> Saturation/1
  Constant10/1 -> Divide3/1
  bat1/1 -> Relational Operator4/1, Scope6/1, Divide2/2
  Saturation/1 -> I_rex 1/1, Scope13/1
  Constant2/1 -> Divide2/1
  Constant3/1 -> Divide2/3

== system HVModAL_Fahrzeugmodell/Energy Manager (Emg)/Battery Control/Driving_Mode/Strategy_Maximiziation_Driving_Range1/Minloss Strategy/Insufficient Energy ==
  SB_BMS_1 : Inport
  SB_BMS_2 : Inport  Port=2
  "SB_BMS_3 " : Inport  Port=3
  "Pload " : Inport  Port=4
  Enable : EnablePort
  Add : Sum
  Add1 : Sum  Inputs=-+
  Bus Selector : BusSelector  OutputSignals=SOC_perc,P_max_charge_10s_W,P_max_discharge_10s_W
  Bus Selector1 : BusSelector  OutputSignals=SOC_perc,P_max_charge_10s_W,P_max_discharge_10s_W
  C_Bat1 : Constant  Value=hvb.Bat1.C_NennZelle
  C_Bat2 : Constant  Value=hvb.Bat2.C_NennZelle
  C_Bat3 : Constant
  C_Bat4 : Constant  Value=0
  C_Bat5 : Constant  Value=0
  Divide : Product  Inputs=*/
  Gain2 : Gain  Gain=100
  Mux1 : Mux  Inputs=3
  "Pack1 cell Number " : Gain  Gain=hvb.Bat1.Num_Zellen_el_par*hvb.Bat1.Num_Zellen_el_ser
  Pack1 cell Number 1 : Gain  Gain=hvb.Bat2.Num_Zellen_el_par*hvb.Bat2.Num_Zellen_el_ser
  Power Limit1 : PowerLimitBlock/Power Limit
  Product : Product
  Product1 : Product
  Saturation : Saturate  UpperLimit=inf  LowerLimit=0.01
  Saturation1 : Saturate  UpperLimit=inf  LowerLimit=0.01
  Terminator : Terminator
  vector_PowerDistribution : Outport
  P_exchange_Master_Slave : Outport  Port=2
  wires:
  "Pload "/1 -> [P_load]
  [P_max_disch_bat3] -> Power Limit1/4
  [P_max_disch_bat2] -> Power Limit1/3
  [P_max_disch_bat1] -> Power Limit1/1
  [P_max_cha_bat1] -> Power Limit1/2
  Bus Selector1/3 -> [P_max_disch_bat2]  "<P_max_discharge_10s_W>"
  Bus Selector1/2 -> [P_max_cha_bat2]  "<P_max_charge_10s_W>"
  Bus Selector/3 -> [P_max_disch_bat1]  "<P_max_discharge_10s_W>"
  Bus Selector/2 -> [P_max_cha_bat1]  "<P_max_charge_10s_W>"
  Power Limit1/2 -> Mux1/2
  Power Limit1/1 -> Mux1/1
  Add1/1 -> Power Limit1/6  "powershare_bat2"
  Divide/1 -> Add1/1, Power Limit1/5  "powershare_bat1"
  [P_load] -> Power Limit1/7
  C_Bat5/1 -> P_exchange_Master_Slave/1
  C_Bat3/1 -> Add1/2
  Add/1 -> Divide/2
  Product1/1 -> Add/2
  Product/1 -> Divide/1, Add/1
  [SOC_Bat2] -> Product1/1
  Pack1 cell Number 1/1 -> Product1/2
  C_Bat2/1 -> Pack1 cell Number 1/1
  "Pack1 cell Number "/1 -> Product/2
  Saturation1/1 -> [SOC_Bat2]
  Saturation/1 -> [SOC_Bat1]
  C_Bat1/1 -> "Pack1 cell Number "/1
  [SOC_Bat1] -> Product/1
  Gain2/1 -> vector_PowerDistribution/1
  Mux1/1 -> Gain2/1
  C_Bat4/1 -> Mux1/3  "powershare_bat3"
  Bus Selector/1 -> Saturation/1  "<SOC_perc>"
  SB_BMS_2/1 -> Bus Selector1/1
  Bus Selector1/1 -> Saturation1/1  "<SOC_perc>"
  SB_BMS_1/1 -> Bus Selector/1
  "SB_BMS_3 "/1 -> Terminator/1

== system HVModAL_Fahrzeugmodell/Energy Manager (Emg)/Battery Control/Driving_Mode/Strategy_Maximiziation_Driving_Range1/Minloss Strategy/Sufficient Energy left ==
  SB_BMS_1 : Inport
  SB_BMS_2 : Inport  Port=2
  "SB_BMS_3 " : Inport  Port=3
  Pload : Inport  Port=4
  Enable : EnablePort
  1-D Lookup Table : Lookup_n-D  NumberOfTableDimensions=1  BreakpointsForDimension1=[20 30 40 50]  Table=[20000 15000 10000 5000]  InternalRulePriority=Speed  RndMeth=Simplest  InputSameDT=on
  Bus Selector : BusSelector  OutputSignals=Ri_Bat_eq,Pack_OCV,P_max_charge_10s_W,P_max_discharge_10s_W,V_Stackvoltage_V,I_Bat_A,SOC_perc
  Bus Selector1 : BusSelector  OutputSignals=Ri_Bat_eq,Pack_OCV,P_max_charge_10s_W,P_max_discharge_10s_W,V_Stackvoltage_V,I_Bat_A,SOC_perc
  Compare To Constant : simulink/Logic and Bit Operations/Compare To Constant  relop=<=  const=50  OutDataTypeStr=boolean
  Logical Operator1 : Logic  Operator=NOT  AllPortsSameDT=off  OutDataTypeStr=boolean
  Logical Operator3 : Logic  AllPortsSameDT=off  OutDataTypeStr=boolean
  Merge : Merge
  Merge1 : Merge
  Minloss Strategy : PowerDistribution_Strategy_MinLoss/Minloss Strategy
  Relational Operator : RelationalOperator  OutDataTypeStr=boolean
  SOC Management : Subsystem
  Terminator : Terminator
  vector_PowerDistribution : Outport
  P_exchange_Master_Slave : Outport  Port=2
  wires:
  Compare To Constant/1 -> Logical Operator3/1
  1-D Lookup Table/1 -> Relational Operator/1
  [SOC_Bat2] -> Compare To Constant/1, 1-D Lookup Table/1
  Bus Selector/1 -> [Ri_Bat1_eq]  "<Ri_Bat_eq>"
  SOC Management/2(P_exchange_Master_Slave) -> Merge1/2
  Minloss Strategy/2 -> Merge1/1
  Merge1/1 -> P_exchange_Master_Slave/1
  [P_max_char_Bat1] -> SOC Management/9(P_max_char_bat1)
  [P_max_disch_Bat2] -> SOC Management/8(P_max_disch_bat2)
  [P_max_char_Bat2] -> Minloss Strategy/9
  [P_max_char_Bat2] -> SOC Management/7(P_max_char_bat2)
  [P_max_char_Bat1] -> Minloss Strategy/7
  [P_max_disch_Bat2] -> Minloss Strategy/8
  [P_max_disch_Bat1] -> Minloss Strategy/6
  [Ri_Bat2_eq] -> SOC Management/3(R2), Minloss Strategy/3  "R2"
  Logical Operator3/1 -> SOC Management/Enable, Logical Operator1/1
  Bus Selector/7 -> [SOC_Bat1]  "<SOC_perc>"
  Bus Selector1/4 -> [P_max_disch_Bat2]  "<P_max_discharge_10s_W>"
  [P_load] -> Relational Operator/2, SOC Management/1(Pload), Minloss Strategy/1  "Pload"
  Logical Operator1/1 -> Minloss Strategy/Enable
  [P_max_disch_Bat1] -> SOC Management/6(P_max_disch_bat1)
  Pload/1 -> [P_load]
  SOC Management/1(vector_PowerDistribution) -> Merge/2
  [OCV_Bat1] -> SOC Management/4(V1), Minloss Strategy/4  "OCV1"
  [OCV_Bat2] -> SOC Management/5(V2), Minloss Strategy/5  "OCV2"
  Merge/1 -> vector_PowerDistribution/1
  [Ri_Bat1_eq] -> SOC Management/2(R1), Minloss Strategy/2  "R1"
  Minloss Strategy/1 -> Merge/1
  Bus Selector/3 -> [P_max_char_Bat1]  "<P_max_charge_10s_W>"
  SB_BMS_2/1 -> Bus Selector1/1
  Bus Selector1/7 -> [SOC_Bat2]  "<SOC_perc>"
  Bus Selector/4 -> [P_max_disch_Bat1]  "<P_max_discharge_10s_W>"
  Bus Selector/2 -> [OCV_Bat1]  "<Pack_OCV>"
  SB_BMS_1/1 -> Bus Selector/1
  Bus Selector1/1 -> [Ri_Bat2_eq]  "<Ri_Bat_eq>"
  Bus Selector/6 -> [I_pack_Bat1]  "<I_Bat_A>"
  Bus Selector1/3 -> [P_max_char_Bat2]  "<P_max_charge_10s_W>"
  Bus Selector1/2 -> [OCV_Bat2]  "<Pack_OCV>"
  Bus Selector/5 -> [V_pack_Bat1]  "<V_Stackvoltage_V>"
  Bus Selector1/5 -> [V_pack_Bat2]  "<V_Stackvoltage_V>"
  "SB_BMS_3 "/1 -> Terminator/1
  Bus Selector1/6 -> [I_pack_Bat2]  "<I_Bat_A>"
  Relational Operator/1 -> Logical Operator3/2

== system HVModAL_Fahrzeugmodell/Traction Inverters (Tri)/Tri1/Thermal Model/Conventional thermal model/Conventional thermal model/Subsystem ==
  note: cross coupling example: Mh to Dh = MOSFET highside to Diode lowside
  Ploss Mh : Inport
  Ploss Dh : Inport  Port=2
  Ploss Ml : Inport  Port=3
  Ploss Dl : Inport  Port=4
  Water Temperature : Inport  Port=5
  Dh to Dh : TransferFcn  Numerator=[TRIname.ThermalModel.conventional.R_th(2,2)]  Denominator=[TRIname.ThermalModel.conventional.R_th(2,2).*TRIname.ThermalModel.conventional.C_th(2,2) 1]
  Dh to Dh1 : TransferFcn  Numerator=[TRIname.ThermalModel.conventional.R_th(2,3)]  Denominator=[TRIname.ThermalModel.conventional.R_th(2,3).*TRIname.ThermalModel.conventional.C_th(2,3) 1]
  Dh to Dh2 : TransferFcn  Numerator=[TRIname.ThermalModel.conventional.R_th(2,4)]  Denominator=[TRIname.ThermalModel.conventional.R_th(2,4).*TRIname.ThermalModel.conventional.C_th(2,4) 1]
  Dh to Mh : TransferFcn  Numerator=[TRIname.ThermalModel.conventional.R_th(2,1)]  Denominator=[TRIname.ThermalModel.conventional.R_th(2,1).*TRIname.ThermalModel.conventional.C_th(2,1) 1]
  Dl to Dh : TransferFcn  Numerator=[TRIname.ThermalModel.conventional.R_th(4,2)]  Denominator=[TRIname.ThermalModel.conventional.R_th(4,2).*TRIname.ThermalModel.conventional.C_th(4,2) 1]
  Dl to Dh1 : TransferFcn  Numerator=[TRIname.ThermalModel.conventional.R_th(4,3)]  Denominator=[TRIname.ThermalModel.conventional.R_th(4,3).*TRIname.ThermalModel.conventional.C_th(4,3) 1]
  Dl to Dh2 : TransferFcn  Numerator=[TRIname.ThermalModel.conventional.R_th(4,4)]  Denominator=[TRIname.ThermalModel.conventional.R_th(4,4).*TRIname.ThermalModel.conventional.C_th(4,4) 1]
  Dl to Mh : TransferFcn  Numerator=[TRIname.ThermalModel.conventional.R_th(4,1)]  Denominator=[TRIname.ThermalModel.conventional.R_th(4,1).*TRIname.ThermalModel.conventional.C_th(4,1) 1]
  Mh to Dh : TransferFcn  Numerator=[TRIname.ThermalModel.conventional.R_th(1,2)]  Denominator=[TRIname.ThermalModel.conventional.R_th(1,2).*TRIname.ThermalModel.conventional.C_th(1,2) 1]
  Mh to Dh1 : TransferFcn  Numerator=[TRIname.ThermalModel.conventional.R_th(1,3)]  Denominator=[TRIname.ThermalModel.conventional.R_th(1,3).*TRIname.ThermalModel.conventional.C_th(1,3) 1]
  Mh to Dh2 : TransferFcn  Numerator=[TRIname.ThermalModel.conventional.R_th(1,4)]  Denominator=[TRIname.ThermalModel.conventional.R_th(1,4).*TRIname.ThermalModel.conventional.C_th(1,4) 1]
  Mh to Mh : TransferFcn  Numerator=[TRIname.ThermalModel.conventional.R_th(1,1)]  Denominator=[TRIname.ThermalModel.conventional.R_th(1,1).*TRIname.ThermalModel.conventional.C_th(1,1) 1]
  Ml to Dh : TransferFcn  Numerator=[TRIname.ThermalModel.conventional.R_th(3,2)]  Denominator=[TRIname.ThermalModel.conventional.R_th(3,2).*TRIname.ThermalModel.conventional.C_th(3,2) 1]
  Ml to Dh1 : TransferFcn  Numerator=[TRIname.ThermalModel.conventional.R_th(3,3)]  Denominator=[TRIname.ThermalModel.conventional.R_th(3,3).*TRIname.ThermalModel.conventional.C_th(3,3) 1]
  Ml to Dh2 : TransferFcn  Numerator=[TRIname.ThermalModel.conventional.R_th(3,4)]  Denominator=[TRIname.ThermalModel.conventional.R_th(3,4).*TRIname.ThermalModel.conventional.C_th(3,4) 1]
  Ml to Mh : TransferFcn  Numerator=[TRIname.ThermalModel.conventional.R_th(3,1)]  Denominator=[TRIname.ThermalModel.conventional.R_th(3,1).*TRIname.ThermalModel.conventional.C_th(3,1) 1]
  Sum{,1..3,5..7,9..13,15} (13 alike) : Sum  Inputs=|++
  Sum14 : Sum  Inputs=++|
  Sum4 : Sum  Inputs=++|
  Sum8 : Sum  Inputs=++|
  T Mh : Outport
  T Dh : Outport  Port=2
  T Ml : Outport  Port=3
  T Dl : Outport  Port=4
  wires:
  Sum/1 -> T Mh/1
  Mh to Mh/1 -> Sum1/1
  Dh to Mh/1 -> Sum1/2
  Ploss Ml/1 -> Ml to Dh2/1, Ml to Dh1/1, Ml to Dh/1, Ml to Mh/1
  Sum1/1 -> Sum2/1
  Ml to Mh/1 -> Sum2/2
  Sum2/1 -> Sum3/1
  Dl to Mh/1 -> Sum3/2
  Sum3/1 -> Sum/1
  Sum4/1 -> T Dh/1
  Mh to Dh/1 -> Sum5/1
  Dh to Dh/1 -> Sum5/2
  Sum5/1 -> Sum6/1
  Ml to Dh/1 -> Sum6/2
  Sum6/1 -> Sum7/1
  Dl to Dh/1 -> Sum7/2
  Sum7/1 -> Sum4/2
  Water Temperature/1 -> Sum8/1, Sum14/1, Sum4/1, Sum/2
  Mh to Dh1/1 -> Sum9/1
  Dh to Dh1/1 -> Sum9/2
  Sum9/1 -> Sum10/1
  Ml to Dh1/1 -> Sum10/2
  Sum10/1 -> Sum11/1
  Dl to Dh1/1 -> Sum11/2
  Sum11/1 -> Sum8/2
  Mh to Dh2/1 -> Sum15/1
  Ploss Mh/1 -> Mh to Dh2/1, Mh to Dh1/1, Mh to Dh/1, Mh to Mh/1
  Dh to Dh2/1 -> Sum15/2
  Ploss Dh/1 -> Dh to Mh/1, Dh to Dh2/1, Dh to Dh1/1, Dh to Dh/1
  Sum15/1 -> Sum12/1
  Ml to Dh2/1 -> Sum12/2
  Sum12/1 -> Sum13/1
  Dl to Dh2/1 -> Sum13/2
  Ploss Dl/1 -> Dl to Dh2/1, Dl to Dh1/1, Dl to Dh/1, Dl to Mh/1
  Sum13/1 -> Sum14/2
  Sum8/1 -> T Ml/1
  Sum14/1 -> T Dl/1

== system HVModAL_Fahrzeugmodell/Traction Inverters (Tri)/Tri1/Thermal Model old/Thermal Junction Model/Leg 1/__InputSSForSFun__ ==
  In1 : Inport
  __UniqueOutportName__1__ : Outport
  wires:
  In1/1 -> __UniqueOutportName__1__/1

== system HVModAL_Fahrzeugmodell/Traction Inverters (Tri)/Tri1/Thermal Model old/Thermal Junction Model/Leg 1/__OutputSSForSFun__ ==
  __UniqueInportName__1__ : Inport
  Out1 : Outport  InitialOutput=0
  wires:
  __UniqueInportName__1__/1 -> Out1/1

== system HVModAL_Fahrzeugmodell/Traction Inverters (Tri)/Tri1/Thermal Model old/Thermal Junction Model/Leg 2/__InputSSForSFun__ ==
  In1 : Inport
  __UniqueOutportName__1__ : Outport
  wires:
  In1/1 -> __UniqueOutportName__1__/1

== system HVModAL_Fahrzeugmodell/Traction Inverters (Tri)/Tri1/Thermal Model old/Thermal Junction Model/Leg 2/__OutputSSForSFun__ ==
  __UniqueInportName__1__ : Inport
  Out1 : Outport  InitialOutput=0
  wires:
  __UniqueInportName__1__/1 -> Out1/1

== system HVModAL_Fahrzeugmodell/Traction Inverters (Tri)/Tri1/Thermal Model old/Thermal Junction Model/Leg 3/__InputSSForSFun__ ==
  In1 : Inport
  __UniqueOutportName__1__ : Outport
  wires:
  In1/1 -> __UniqueOutportName__1__/1

== system HVModAL_Fahrzeugmodell/Traction Inverters (Tri)/Tri1/Thermal Model old/Thermal Junction Model/Leg 3/__OutputSSForSFun__ ==
  __UniqueInportName__1__ : Inport
  Out1 : Outport  InitialOutput=0
  wires:
  __UniqueInportName__1__/1 -> Out1/1

== system HVModAL_Fahrzeugmodell/Energy Manager (Emg)/Battery Control/Driving_Mode/Range_extender 2/dynamic/power estimination /mapping1 ==
  P_max_ch_W_Bat1 : Inport
  P_max_Disch_W_Bat1 : Inport  Port=2
  Gain : Gain  Gain=-1
  P_LB_Bat1 : Outport
  P_UB_Bat1 : Outport  Port=2
  wires:
  Gain/1 -> P_LB_Bat1/1
  P_max_ch_W_Bat1/1 -> Gain/1
  P_max_Disch_W_Bat1/1 -> P_UB_Bat1/1
